simulink model "perfusion"  (Simulink 6.6)
settings: Solver=ode45  StartTime=0.0  StopTime=24  MaxStep=10  RelTol=1e-3
libraries: simulink x4
settings Model: Creator=asuri  LastModifiedBy=school  ExtModeAutoUpdateStatusClock=off
settings SolverCC: ZeroCrossControl=EnableAll
settings DataIOCC: SaveOutput=off  SaveTime=off
settings OptimizationCC: BooleanDataType=off  InlineInvariantSignals=on
settings DebuggingCC: AlgebraicLoopMsg=error  SignalResolutionControl=TryResolveAllWithWarning  SolverPrmCheckMsg=none  MultiTaskDSMMsg=warning  MultiTaskCondExecSysMsg=none  InvalidFcnCallConnMsg=warning  StrictBusMsg=None
settings RTWCC: IncludeERTFirstTime=on

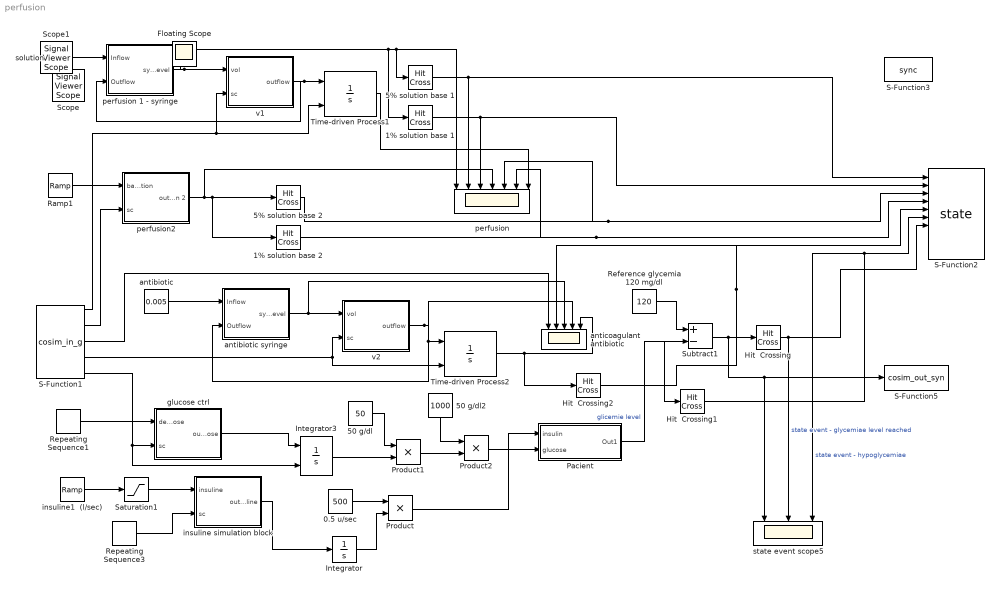
== system perfusion ==
  "0.5 u/sec " : Constant  Value=500
  1% solution base 1 : HitCross  HitCrossingOffset=0.075  HitCrossingDirection=falling  ZeroCross=off
  1% solution base 2 : HitCross  HitCrossingOffset=5  HitCrossingDirection=falling  ZeroCross=off
  5% solution base 1 : HitCross  HitCrossingOffset=0.1  HitCrossingDirection=falling  ZeroCross=off
  5% solution base 2 : HitCross  HitCrossingOffset=25  HitCrossingDirection=falling  ZeroCross=off
  50 g/dl : Constant  Value=50
  50 g/dl2 : Constant  Orientation=down  Value=1000
  Hit  Crossing : HitCross
  Hit  Crossing1 : HitCross  HitCrossingOffset=60  HitCrossingDirection=falling  ZeroCross=off
  Hit  Crossing2 : HitCross  HitCrossingOffset=0.2  HitCrossingDirection=rising  ZeroCross=off
  Integrator : Integrator
  Integrator3 : Integrator  ExternalReset=either
  Pacient : Subsystem
  Product : Product  RndMeth=Zero
  Product1 : Product  RndMeth=Zero
  Product2 : Product  RndMeth=Zero
  Ramp1 : simulink/Sources/Ramp  SystemSampleTime=-1  slope=-35  start=14.2  X0=500
  "Reference glycemia 120 mg/dl " : Constant  Value=120
  Repeating Sequence1 : simulink/Sources/Repeating Sequence  SystemSampleTime=-1  rep_seq_t=[0 1]  rep_seq_y=[0 0.001]
  Repeating Sequence3 : simulink/Sources/Repeating Sequence  SystemSampleTime=-1  rep_seq_t=[0 1 2 3 4 5 6 7 8 9 10 11 12 13 14 15 16 17 18 19 20 21 22 23]  rep_seq_y=[0 0 0 0 0 0 0 0 0 0 0 0 0 0 0 0 0 0 0 1 0 0 0 0]
  S-Function1 : S-Function  Priority=0  FunctionName=cosim_in_g  Parameters=NpIn  mask{NpIn=5}
      mask prompts: NpIn "Number of input ports :"
      mask help: Simulink input ports number.
  S-Function2 : S-Function  FunctionName=state  Parameters=NS  mask{NS=10}
      mask prompts: NS "Number Of Input state events"
      mask help: Specify the number of input state events. It must be less than 10
  S-Function3 : S-Function  FunctionName=sync
  S-Function5 : S-Function  Priority=16  FunctionName=cosim_out_syn  Parameters=NoutPort  mask{NoutPort=1}
      mask prompts: NoutPort "Number of output ports :"
      mask help: 1. Simulink output ports number.
  Saturation1 : Saturate  UpperLimit=0.500  LowerLimit=1e-5
  Subtract1 : Sum  Inputs=+-  OutScaling=2^-10
  Time-driven Process1 : Integrator  ExternalReset=either
  Time-driven Process2 : Integrator  ExternalReset=either
  antibiotic : Constant  Value=0.005
  antibiotic syringe : Subsystem
  anticoagulant antibiotic : Scope  NumInputPorts=5
      settings: Orientation=down  TimeRange=25  YMin=-5~-80~-5~-5~-5  YMax=5~60~5~5~5  SaveName=ScopeData6
  glucose ctrl : Subsystem
  insuline simulation block : Subsystem
  insuline1  (l/sec) : simulink/Sources/Ramp  SystemSampleTime=-1  slope=1e-4/3600  start=0  X0=0
  perfusion : Scope  NumInputPorts=7
      settings: Orientation=down  YMin=119.89~-0.02~-5~0~0~0~-5  YMax=120.01~0.11~5~510~1~1~5  SaveName=ScopeData7
  perfusion 1 - syringe : Subsystem
  perfusion2 : Subsystem
  solution : Constant  Value=0.05
  state event scope5 : Scope  NumInputPorts=3
      settings: Orientation=down  YMin=119.89~-0.02~-5  YMax=120.01~0.11~5  SaveName=ScopeData9
  v1 : Subsystem
  v2 : Subsystem
  Floating Scope : Scope
      settings: Floating=on
  Scope : SignalViewerScope  IOType=viewer  RefreshTime=0.035000
  Scope1 : SignalViewerScope  IOType=viewer  ZoomMode=xonly  RefreshTime=0.035000
      settings: YMin=0  YMax=4
  wires:
  Repeating Sequence1/1 -> glucose ctrl/1(debit glucose)
  50 g/dl/1 -> Product1/1
  Integrator3/1 -> Product1/2
  glucose ctrl/1(outflow glucose) -> Integrator3/1
  Subtract1/1 -> Hit  Crossing/1, S-Function5/1, state event scope5/1
  "Reference glycemia 120 mg/dl "/1 -> Subtract1/1
  Pacient/1(Out1) -> Hit  Crossing1/1, Subtract1/2  "glicemie level"
  Product2/1 -> Pacient/2(glucose)
  Product1/1 -> Product2/2
  1% solution base 1/1 -> S-Function2/2, perfusion/3
  5% solution base 2/1 -> S-Function2/3, perfusion/5
  1% solution base 2/1 -> S-Function2/4, perfusion/6
  Hit  Crossing/1 -> S-Function2/7, state event scope5/2  "state event - glycemiae level reached"
  Hit  Crossing1/1 -> state event scope5/3, S-Function2/6  "state event - hypoglycemiae"
  S-Function1/3 -> anticoagulant antibiotic/1
  S-Function1/5 -> Integrator3/2, glucose ctrl/2(sc)
  5% solution base 1/1 -> perfusion/2, S-Function2/1
  perfusion2/1("output solution 2 ") -> 5% solution base 2/1, 1% solution base 2/1, perfusion/4
  50 g/dl2/1 -> Product2/1
  insuline1  (l/sec)/1 -> Saturation1/1
  Saturation1/1 -> insuline simulation block/1(insuline)
  insuline simulation block/1(outflow insuline) -> Integrator/1
  "0.5 u/sec "/1 -> Product/1
  Integrator/1 -> Product/2
  Product/1 -> Pacient/1(insulin)
  Repeating Sequence3/1 -> insuline simulation block/2(sc)
  antibiotic syringe/1(syringe level) -> v2/1(vol), anticoagulant antibiotic/3
  v2/1(outflow) -> antibiotic syringe/2(Outflow), Time-driven Process2/1, anticoagulant antibiotic/4
  Hit  Crossing2/1 -> S-Function2/5, anticoagulant antibiotic/2
  antibiotic/1 -> antibiotic syringe/1(Inflow)
  S-Function1/2 -> perfusion2/2(sc)
  Ramp1/1 -> perfusion2/1(base solution)
  v1/1(outflow) -> perfusion 1 - syringe/2(Outflow), Time-driven Process1/1
  perfusion 1 - syringe/1(syringe level) -> v1/1(vol), perfusion/1, 5% solution base 1/1, 1% solution base 1/1
  solution/1 -> perfusion 1 - syringe/1(Inflow)
  Time-driven Process1/1 -> perfusion/7
  S-Function1/1 -> v1/2(sc), Time-driven Process1/2
  Time-driven Process2/1 -> anticoagulant antibiotic/5, Hit  Crossing2/1
  S-Function1/4 -> v2/2(sc), Time-driven Process2/2

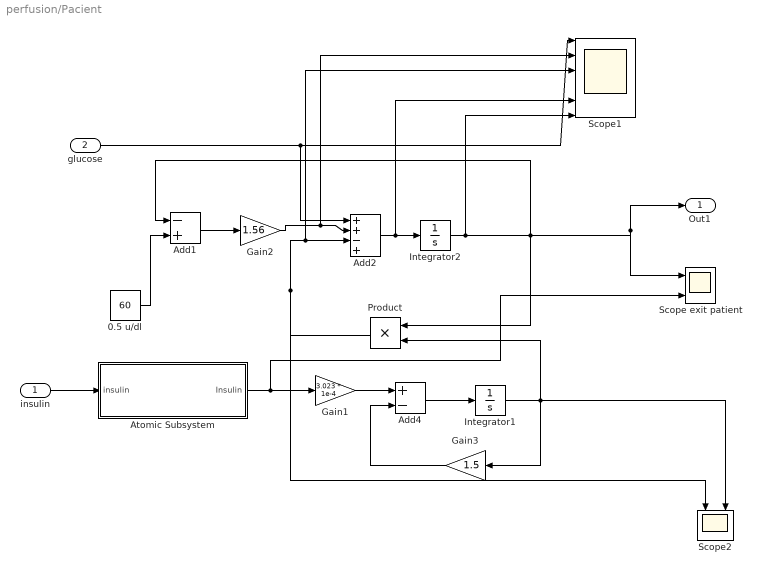
== system perfusion/Pacient ==
  insulin : Inport
  glucose : Inport  Port=2
  "0.5 u/dl " : Constant  Value=60
  Add1 : Sum  Inputs=-+  OutScaling=2^-10
  Add2 : Sum  Inputs=++-+  OutScaling=2^-10
  Add4 : Sum  Inputs=+-  OutScaling=2^-10
  Atomic Subsystem : Subsystem  TreatAsAtomicUnit=on
  Gain1 : Gain  Gain=3.023 * 1e-4
  Gain2 : Gain  Gain=1.56
  Gain3 : Gain  Orientation=left  Gain=1.5
  Integrator1 : Integrator
  Integrator2 : Integrator  InitialCondition=270
  Product : Product  Orientation=left  RndMeth=Zero
  Scope exit patient : Scope  NumInputPorts=2
      settings: TimeRange=25  YMin=118~-8.67362e-019  YMax=120.25~0.0175  SaveName=ScopeData3
  Scope1 : Scope  NumInputPorts=6
      settings: YMin=-1~-5~-5~-5~-5~-5  YMax=1~5~5~5~5~5  SaveName=ScopeData2
  Scope2 : Scope  NumInputPorts=2
      settings: Orientation=down  YMin=48~22  YMax=54.5~28.5  SaveName=ScopeData4
  Out1 : Outport
  wires:
  Add1/1 -> Gain2/1
  Add2/1 -> Integrator2/1, Scope1/5
  Integrator2/1 -> Add1/1, Product/1, Out1/1, Scope exit patient/1, Scope1/6
  Product/1 -> Scope2/1, Add2/3, Scope1/3
  Gain1/1 -> Add4/1
  Add4/1 -> Integrator1/1
  Integrator1/1 -> Gain3/1, Scope2/2, Product/2
  Gain3/1 -> Add4/2
  glucose/1 -> Add2/1, Scope1/1
  insulin/1 -> Atomic Subsystem/1(insulin)
  Atomic Subsystem/1(Insulin) -> Gain1/1, Scope exit patient/2
  Gain2/1 -> Add2/2, Scope1/2
  "0.5 u/dl "/1 -> Add1/2

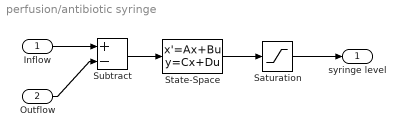
== system perfusion/antibiotic syringe ==
  Inflow : Inport
  Outflow : Inport  Port=2
  Saturation : Saturate  UpperLimit=100  LowerLimit=0
  State-Space : StateSpace  A=0  B=0.5  C=0.5  D=0  X0=3
  Subtract : Sum  Inputs=+-  OutScaling=2^-10
  syringe level : Outport
  wires:
  Subtract/1 -> State-Space/1
  State-Space/1 -> Saturation/1
  Inflow/1 -> Subtract/1
  Saturation/1 -> syringe level/1
  Outflow/1 -> Subtract/2

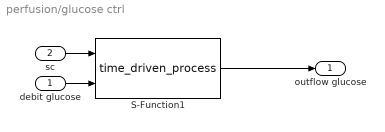
== system perfusion/glucose ctrl ==
  debit glucose : Inport
  sc : Inport  Port=2
  S-Function1 : S-Function  FunctionName=time_driven_process  Parameters=debitMax, debitMin  mask{debitMax=500, debitMin=0}
      mask prompts: debitMax "OutFlowMax"; debitMin "OutFlowMin"
  outflow glucose : Outport
  wires:
  S-Function1/1 -> outflow glucose/1
  sc/1 -> S-Function1/1
  debit glucose/1 -> S-Function1/2

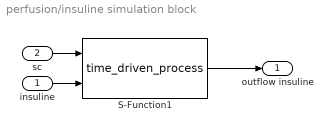
== system perfusion/insuline simulation block ==
  insuline : Inport
  sc : Inport  Port=2
  S-Function1 : S-Function  FunctionName=time_driven_process  Parameters=debitMax, debitMin  mask{debitMax=0.5, debitMin=0}
      mask prompts: debitMax "OutFlowMax"; debitMin "OutFlowMin"
  outflow insuline : Outport
  wires:
  S-Function1/1 -> outflow insuline/1
  sc/1 -> S-Function1/1
  insuline/1 -> S-Function1/2

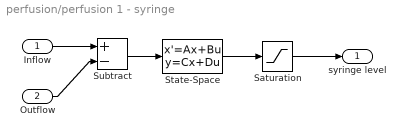
== system perfusion/perfusion 1 - syringe ==
  Inflow : Inport
  Outflow : Inport  Port=2
  Saturation : Saturate  UpperLimit=100  LowerLimit=0
  State-Space : StateSpace  A=0  B=0.5  C=0.5  D=0  X0=3
  Subtract : Sum  Inputs=+-  OutScaling=2^-10
  syringe level : Outport
  wires:
  Subtract/1 -> State-Space/1
  State-Space/1 -> Saturation/1
  Inflow/1 -> Subtract/1
  Saturation/1 -> syringe level/1
  Outflow/1 -> Subtract/2

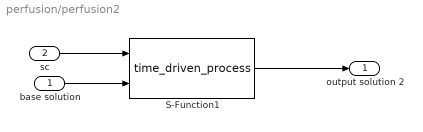
== system perfusion/perfusion2 ==
  base solution : Inport
  sc : Inport  Port=2
  S-Function1 : S-Function  FunctionName=time_driven_process  Parameters=debitMax, debitMin  mask{debitMax=500, debitMin=0}
      mask prompts: debitMax "OutFlowMax"; debitMin "OutFlowMin"
  "output solution 2 " : Outport
  wires:
  sc/1 -> S-Function1/1
  base solution/1 -> S-Function1/2
  S-Function1/1 -> "output solution 2 "/1

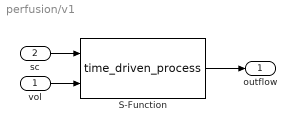
== system perfusion/v1 ==
  vol : Inport
  sc : Inport  Port=2
  S-Function : S-Function  FunctionName=time_driven_process  Parameters=debitMax, debitMin  mask{debitMax=0.003, debitMin=0.003}
      mask prompts: debitMax "OutFlowMax"; debitMin "OutFlowMin"
  outflow : Outport
  wires:
  S-Function/1 -> outflow/1
  sc/1 -> S-Function/1
  vol/1 -> S-Function/2

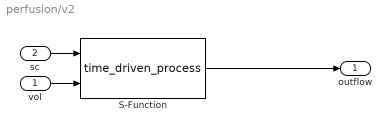
== system perfusion/v2 ==
  vol : Inport
  sc : Inport  Port=2
  S-Function : S-Function  FunctionName=time_driven_process  Parameters=debitMax, debitMin  mask{debitMax=0.003, debitMin=0.003}
      mask prompts: debitMax "OutFlowMax"; debitMin "OutFlowMin"
  outflow : Outport
  wires:
  sc/1 -> S-Function/1
  vol/1 -> S-Function/2
  S-Function/1 -> outflow/1

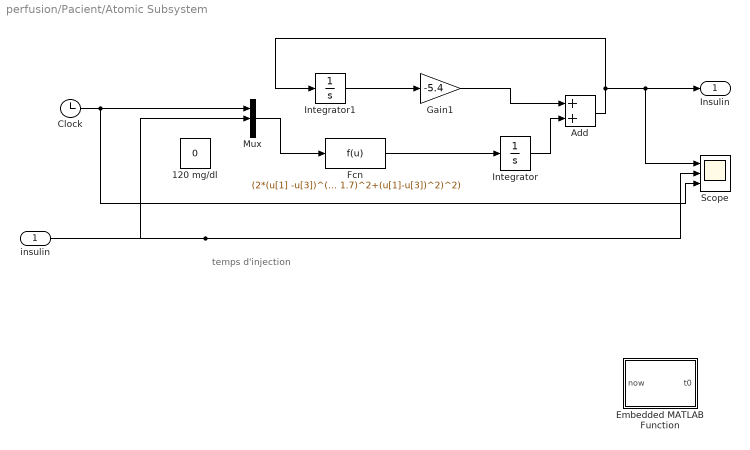
== system perfusion/Pacient/Atomic Subsystem ==
  note: temps d'injection
  insulin : Inport
  120 mg/dl : Constant  Value=0
  Add : Sum  OutScaling=2^-10
  Clock : Clock
      settings: Decimation=10
  Embedded MATLAB Function : Stateflow chart
  Fcn : Fcn  Expr=(2*(u[1] -u[3])^(2-1)*u[2] * (0.05*u[2] + 1.7)^2)/(120*( (0.05*u[2] + 1.7)^2+(u[1]-u[3])^2)^2)
  Gain1 : Gain  Gain=-5.4
  Integrator : Integrator
  Integrator1 : Integrator
  Mux : Mux  Inputs=3
  Scope : Scope  NumInputPorts=3
      settings: YMin=-1e-008~0~-5  YMax=1.2e-007~9.5e+010~5
  Insulin : Outport
  wires:
  Fcn/1 -> Integrator/1
  Integrator/1 -> Add/2
  Gain1/1 -> Add/1
  Add/1 -> Scope/1, Insulin/1, Integrator1/1
  insulin/1 -> Mux/2, Scope/2
  Mux/1 -> Fcn/1
  Clock/1 -> Mux/1, Scope/3
  Integrator1/1 -> Gain1/1

== matlab function Pacient/Atomic Subsystem/Embedded MATLAB Function ==
  data: now input inherited; t0 output inherited
function t0 = fcn(now)
% This block supports an embeddable subset of the MATLAB language.
% See the help menu for details. 

if now < 3600*1
    t0 = 0;
else
    t0 = 3600*1;
end
